simulink model "ParmTests_v1"  (Simulink 7.5)
settings: Solver=ode45  StartTime=0.0  StopTime=10.0  RelTol=1e-3
settings Model: Creator=Robert  LastModifiedBy=Robert

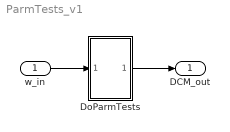
== system ParmTests_v1 ==
  w_in : Inport  OutDataType=fixdt(1, 16)  OutScaling=2^0
  DoParmTests : Subsystem
  DCM_out : Outport  OutDataType=fixdt(1, 16)  OutScaling=2^0
  wires:
  DoParmTests/1(Out1) -> DCM_out/1
  w_in/1 -> DoParmTests/1(In1)

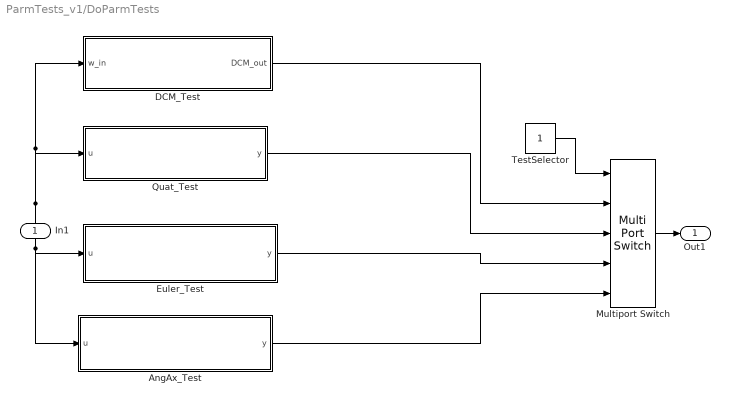
== system ParmTests_v1/DoParmTests ==
  In1 : Inport
  AngAx_Test : Stateflow chart  TreatAsAtomicUnit=on
  DCM_Test : Stateflow chart  TreatAsAtomicUnit=on
  Euler_Test : Stateflow chart  TreatAsAtomicUnit=on
  Multiport Switch : MultiPortSwitch  Inputs=4  zeroidx=off  OutDataType=fixdt(1, 16)  OutScaling=2^0
  Quat_Test : Stateflow chart  TreatAsAtomicUnit=on
  TestSelector : Constant  OutDataType=fixdt(1, 16)  OutScaling=2^0
  Out1 : Outport
  wires:
  DCM_Test/1(DCM_out) -> Multiport Switch/2
  Quat_Test/1(y) -> Multiport Switch/3
  Euler_Test/1(y) -> Multiport Switch/4
  AngAx_Test/1(y) -> Multiport Switch/5
  TestSelector/1 -> Multiport Switch/1
  In1/1 -> DCM_Test/1(w_in), Quat_Test/1(u), Euler_Test/1(u), AngAx_Test/1(u)
  Multiport Switch/1 -> Out1/1

== matlab function DoParmTests/Quat_Test ==
  data: u input double; y output double
function y = fcn(u)
%#eml

y = u;

== matlab function DoParmTests/Euler_Test ==
  data: u input double; y output double
function y = fcn(u)
%#eml

y = u;

== matlab function DoParmTests/AngAx_Test ==
  data: u input double; y output double
function y = fcn(u)
%#eml

y = u;

== matlab function DoParmTests/DCM_Test ==
  data: w_in input double; DCM_out output double
function DCM_out = DCM_Test(w_in)
%#eml
% Embedded Matlab code to handle the DCM attitude propagation
% PARAMETERS
% w_in - gyro inputs, p q r
% RETVAL
% DCM_out - 3x3 matrix of attitude representation

persistent p; 
persistent q;
persistent r;
persistent DCM;

SampleT = apSampleTime;

TEST_FWDEULERCONST = 1;
TEST_FWDEULERTRAP  = 2;
TEST_MEXPCONSTPREV = 3;
TEST_MEXPCONSTCURR = 4;
TEST_MEXPTRAP      = 5;
TEST_MEXPBAR       = 6;
test_case          = TEST_FWDEULERCONST;

% Indices
% pqr
wcurr  = 3;
wprev  = 2;
wprev2 = 1;

% dcm
rcurr = 2;
rprev = 1;

% PERSISTENT VARIABLES:  Set up arrays to maintain 3 time values of each angular velocity reading.
% Before initialization:  pqr = [ 0       0        0   ]
% After initialization:   pqr = [ pqr(1) pqr(1) pqr(1) ], where pqr(1) == w_in( 1/2/3 )
% 2nd step:               pqr = [ pqr(1) pqr(1) pqr(2) ]
% 3rd step:               pqr = [ pqr(1) pqr(2) pqr(3) ]
% 4th step:               pqr = [ pqr(2) pqr(3) pqr(4) ]
% ...
% Same setup with DCM, but only 2 placeholders:  DCM = [ DCM(1) DCM(1) ]

% Update the pqr arrays appropriately
if( isempty( p ) ) % init array
    p = w_in(1) * ones( 3, 1 );
else % shift left and insert new value
    p(wprev2) = p(wprev);
    p(wprev ) = p(wcurr);
    p(wcurr ) = w_in(1);
end

if( isempty( q ) )
    q = w_in(2) * ones( 3, 1 );
else % shift left and insert new value
    q(wprev2) = q(wprev);
    q(wprev ) = q(wcurr);
    q(wcurr ) = w_in(2);    
end

if( isempty( r ) )
    r = w_in(3) * ones( 3, 1 );
else % shift left and insert new value
    r(wprev2) = r(wprev);
    r(wprev ) = r(wcurr);
    r(wcurr ) = w_in(3);      
end

if( isempty( DCM ) )
    DCM = zeros( 3, 3, 2 );  % Keep current and previous DCM
    DCM(:,:,rprev) = R0;
else
    DCM(:,:,rprev) = DCM(:,:,rcurr); % shift left.  rcurr will be updated later
end

% Propagation step
switch test_case
    case TEST_FWDEULERCONST
        dOmegaX_c = pqr2OmegaX_dcm( p(wprev), q(wprev), r(wprev) );
        dcm_dot_c = Rdot( dOmegaX_c, DCM(:,:,rprev)); 
        DCM(:,:,rcurr) = FwdEuler( dcm_dot_c, SampleT, DCM(:,:,rprev) );
        
    case TEST_FWDEULERTRAP
        p_t = (1/2)*( p(wcurr) + p(wprev) );
        q_t = (1/2)*( q(wcurr) + q(wprev) );
        r_t = (1/2)*( r(wcurr) + r(wprev) );
        dOmegaX_t = pqr2OmegaX_dcm( p_t, q_t, r_t );
        dcm_dot_t = Rdot( dOmegaX_t, DCM(:,:,rprev)); 
        DCM(:,:,rcurr) = FwdEuler( dcm_dot_t, SampleT, DCM(:,:,rprev) );        
        
    case TEST_MEXPCONSTPREV
        p_cp = p(wprev);
        q_cp = q(wprev);
        r_cp = r(wprev);
        dOmegaX_cp = pqr2OmegaX_dcm( p_cp, q_cp, r_cp );
        DCM(:,:,rcurr) = RMe_Int3( dOmegaX_cp, DCM(:,:,rprev), SampleT );         
        
    case TEST_MEXPCONSTCURR
        p_cc = p(wcurr);
        q_cc = q(wcurr);
        r_cc = r(wcurr);
        dOmegaX_cc = pqr2OmegaX_dcm( p_cc, q_cc, r_cc );
        DCM(:,:,rcurr) = RMe_Int3( dOmegaX_cc, DCM(:,:,rprev), SampleT );         
        
    case TEST_MEXPTRAP
        p_t = (1/2)*( p(wcurr) + p(wprev) );
        q_t = (1/2)*( q(wcurr) + q(wprev) );
        r_t = (1/2)*( r(wcurr) + r(wprev) );
        dOmegaX_met = pqr2OmegaX_dcm( p_t, q_t, r_t );
        DCM(:,:,rcurr) = RMe_Int3( dOmegaX_met, DCM(:,:,rprev), SampleT ); 
        
    case TEST_MEXPBAR
        OxCurr  = pqr2OmegaX_dcm( p( wcurr  ), q( wcurr  ), r( wcurr  ));
        OxPrev  = pqr2OmegaX_dcm( p( wprev  ), q( wprev  ), r( wprev  ));
        OxPrev2 = pqr2OmegaX_dcm( p( wprev2 ), q( wprev2 ), r( wprev2 ));

        % For the first 2 timesteps, Odot/Oddot/OmBar == 0.
        Odot  = OmegaDot( OxCurr, OxPrev2, SampleT );
        Oddot = OmegaDDot( OxCurr, OxPrev, OxPrev2, SampleT );
        OmBar = OmegaBar( OxPrev, Odot, Oddot, SampleT );

        DCM(:,:,rcurr) = RMe_Int3( OmBar, DCM(:,:,rprev), SampleT );    

end  %switch test_case

DCM_out = DCM(:,:,rcurr);
